simulink model "rlcCircuit"  (R2021a)
settings: Solver=ode4  StartTime=0.0  StopTime=0.1  FixedStep=1e-7  RelTol=1e-3
settings Model: Creator=Asus  LastModifiedBy=Asus

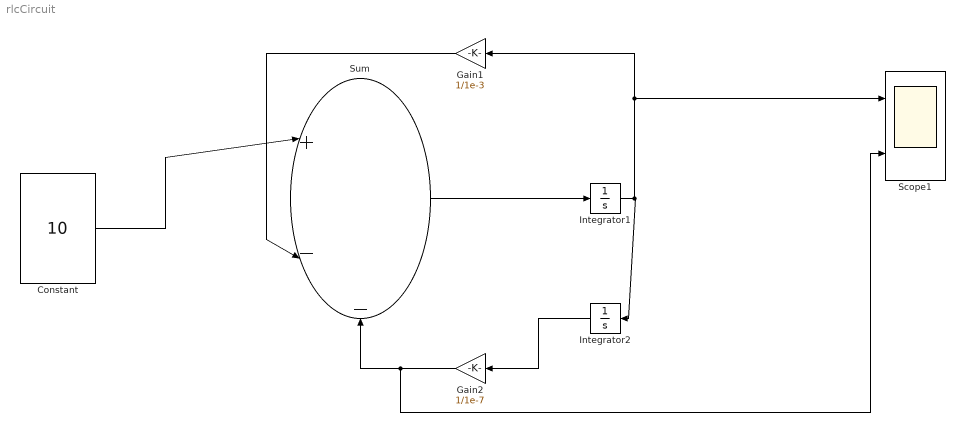
== system rlcCircuit ==
  Constant : Constant  Value=10
  Gain1 : Gain  Gain=1/1e-3
  Gain2 : Gain  Gain=1/1e-7
  Integrator1 : Integrator
  Integrator2 : Integrator
  Scope1 : Scope  NumInputPorts=2
  Sum : Sum  Inputs=|+--
  wires:
  Constant/1 -> Sum/1
  Gain1/1 -> Sum/2
  Sum/1 -> Integrator1/1
  Integrator1/1 -> Gain1/1, Scope1/1, Integrator2/1
  Integrator2/1 -> Gain2/1
  Gain2/1 -> Sum/3, Scope1/2
